simulink model "GuidanceSimV3"  (R2024b)
settings: Solver=VariableStepAuto  StartTime=0.0  StopTime=inf  FixedStep=0.05  RelTol=1e-3
values from neighbouring files (symbols this model uses):
  a_max = 10    [GuidanceSimParams.m]
  a_min = -10    [GuidanceSimParams.m]
  gM = asin(2/3*sin(gT-LOS))+LOS    [GuidanceSimParams.m]
  N = 3.5    [GuidanceSimParams.m]
  Rlethal = 1    [GuidanceSimParams.m]
  RM = [xM;zM]    [GuidanceSimParams.m]
  RT = [xT;zT]    [GuidanceSimParams.m]
  Vcinit = MS*cos(gM-LOS)-TS*cos(gT-LOS)    [GuidanceSimParams.m]
  VM = [600*cos(gM),-600*sin(gM)]    [GuidanceSimParams.m]
  VT = [400*cos(gT),-400*sin(gT)]    [GuidanceSimParams.m]
  Wn_hom = 7    [GuidanceSimParams.m]
undefined symbols (not defined in the file or in its folder): eta, type
libraries: simulink_extras x2, simulink x2, aerolibanim x1
settings Model: Creator=Ameya  LastModifiedBy=Ameya
settings SolverCC: EnableFixedStepZeroCrossing=on

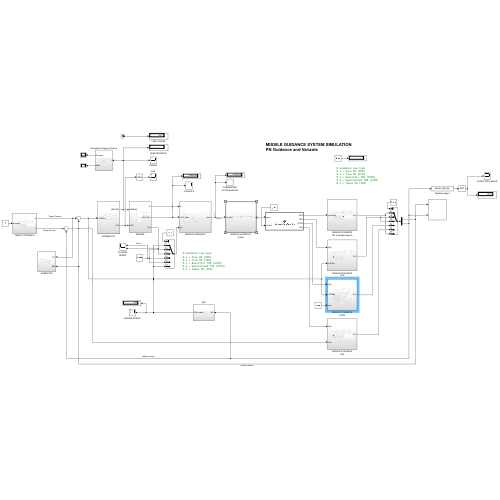
[thumbnail: Simulink's stored preview of the top-level diagram]
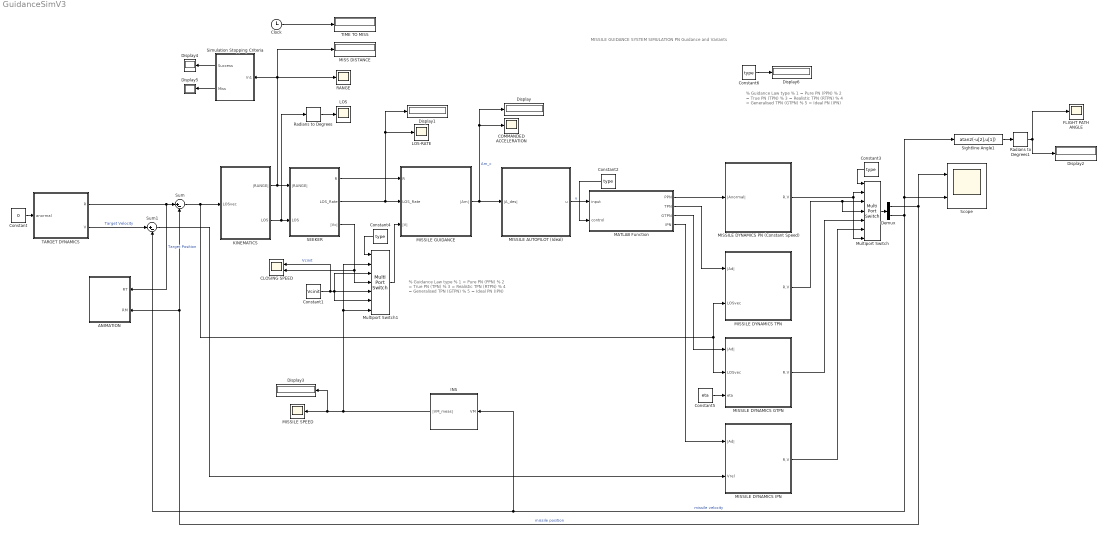
== system GuidanceSimV3 ==
  note: % Guidance Law type
      | % 1 = Pure PN (PPN)
      | % 2 = True PN (TPN)
      | % 3 = Realistic TPN (RTPN)
      | % 4 = Generalised TPN (GTPN)
      | % 5 = Ideal PN (IPN)
  note: MISSILE GUIDANCE SYSTEM SIMULATION
      | PN Guidance and Variants
  note: % Guidance Law type
      | % 1 = Pure PN (PPN)
      | % 2 = True PN (TPN)
      | % 3 = Realistic TPN (RTPN)
      | % 4 = Generalised TPN (GTPN)
      | % 5 = Ideal PN (IPN)
  ANIMATION : Subsystem
  CLOSING SPEED : Scope  NumInputPorts=2
  COMMANDED ACCELERATION : Scope
  Clock : Clock
  Constant : Constant  Value=0
  Constant1 : Constant  Value=Vcinit
  Constant{2..4,6} (4 alike) : Constant  Value=type
  Constant5 : Constant  Value=eta
  Demux : Demux  Outputs=2
  Display{,1..6} (7 alike) : Display
  FLIGHT PATH ANGLE : Scope
  INS : Subsystem
  KINEMATICS : Subsystem
  LOS : Scope
  LOS-RATE : Scope
  MATLAB Function : MATLAB Function  TreatAsAtomicUnit=on
  MISS DISTANCE : Display
  MISSILE AUTOPILOT (Ideal) : Subsystem
  MISSILE DYNAMICS GTPN : Subsystem
  MISSILE DYNAMICS IPN : Subsystem
  MISSILE DYNAMICS PN (Constant Speed) : Subsystem
  MISSILE DYNAMICS TPN : Subsystem
  MISSILE GUIDANCE : Subsystem
  MISSILE SPEED : Scope
  Multiport Switch : MultiPortSwitch  Inputs=5  DataPortForDefault=Additional data port  SaturateOnIntegerOverflow=off  InputSameDT=off
  Multiport Switch1 : MultiPortSwitch  Inputs=5  DataPortForDefault=Additional data port  SaturateOnIntegerOverflow=off  InputSameDT=off
  RANGE : Scope
  Radians to Degrees : simulink_extras/Transformations/Radians to Degrees
  Radians to Degrees1 : simulink_extras/Transformations/Radians to Degrees
  SEEKER : Subsystem
  Scope : Scope  NumInputPorts=2
  Sightline Angle1 : Fcn  Expr=atan2(-u[2],u[1])
  Simulation Stopping Criteria : Subsystem
  Sum : Sum  Inputs=|+-
  Sum1 : Sum  Inputs=|+-
  TARGET DYNAMICS : Subsystem
  TIME TO MISS : Display
  wires:
  MISSILE GUIDANCE/1(|Am|) -> COMMANDED ACCELERATION/1, Display/1, MISSILE AUTOPILOT (Ideal)/1(|A_des|)  "Am_c"
  Constant/1 -> TARGET DYNAMICS/1(anormal)
  Radians to Degrees/1 -> LOS/1
  INS/1(|VM_meas|) -> Display3/1, MISSILE SPEED/1, Multiport Switch1/7, Multiport Switch1/2
  TARGET DYNAMICS/1(R) -> ANIMATION/1(RT), Sum/1  "Target Position"
  Sum/1 -> MISSILE DYNAMICS TPN/2(LOSvec), MISSILE DYNAMICS GTPN/2(LOSvec), KINEMATICS/1(LOSvec)
  KINEMATICS/1(|RANGE|) -> Simulation Stopping Criteria/1(In1), RANGE/1, MISS DISTANCE/1, SEEKER/1(|RANGE|)
  KINEMATICS/2(LOS) -> Radians to Degrees/1, SEEKER/2(LOS)
  SEEKER/2(LOS_Rate) -> Display1/1, LOS-RATE/1, MISSILE GUIDANCE/2(LOS_Rate)
  SEEKER/1(R) -> MISSILE GUIDANCE/1(R)
  Sightline Angle1/1 -> Radians to Degrees1/1
  Radians to Degrees1/1 -> FLIGHT PATH ANGLE/1, Display2/1
  Simulation Stopping Criteria/1(Success) -> Display4/1
  Simulation Stopping Criteria/2(Miss) -> Display5/1
  MISSILE AUTOPILOT (Ideal)/1(u) -> MATLAB Function/1(input)  "u"
  Constant2/1 -> MATLAB Function/2(control)
  MATLAB Function/1(PPN) -> MISSILE DYNAMICS PN (Constant Speed)/1(|Anormal|)
  MATLAB Function/2(TPN) -> MISSILE DYNAMICS TPN/1(|Ad|)
  MATLAB Function/3(GTPN) -> MISSILE DYNAMICS GTPN/1(|Ad|)
  MISSILE DYNAMICS PN (Constant Speed)/1(R,V) -> Multiport Switch/7, Multiport Switch/2
  MISSILE DYNAMICS TPN/1(R,V) -> Multiport Switch/4, Multiport Switch/3
  MISSILE DYNAMICS GTPN/1(R,V) -> Multiport Switch/5
  Constant3/1 -> Multiport Switch/1
  Multiport Switch/1 -> Demux/1
  Demux/1 -> Sum/2, ANIMATION/2(RM), Scope/1  "missile position"
  Demux/2 -> INS/1(VM), Sum1/2, Sightline Angle1/1, Scope/2  "missile velocity"
  MATLAB Function/4(IPN) -> MISSILE DYNAMICS IPN/1(|Ad|)
  TARGET DYNAMICS/2(V) -> Sum1/1  "Target Velocity"
  Sum1/1 -> MISSILE DYNAMICS IPN/2(Vrel)
  MISSILE DYNAMICS IPN/1(R,V) -> Multiport Switch/6
  Multiport Switch1/1 -> MISSILE GUIDANCE/3(|V|)
  Constant1/1 -> CLOSING SPEED/1, Multiport Switch1/3, Multiport Switch1/6, Multiport Switch1/5  "Vcinit"
  SEEKER/3(|Vc|) -> CLOSING SPEED/2, Multiport Switch1/4
  Constant4/1 -> Multiport Switch1/1
  Constant5/1 -> MISSILE DYNAMICS GTPN/3(eta)
  Clock/1 -> TIME TO MISS/1
  Constant6/1 -> Display6/1

== system GuidanceSimV3/ANIMATION ==
  RT : Inport
  RM : Inport  Port=2
  3DoF Animation1 : aerolibanim/3DoF Animation  u1=[0 5000 -2000 2000 -5050 -3]  u2=0.05  u3=1  u5=Fly alongside  u6=[2000 500 -3150]  u7=10  u8=off
  Constant1 : Constant  Value=gM
  wires:
  Constant1/1 -> 3DoF Animation1/3
  RT/1 -> 3DoF Animation1/1
  RM/1 -> 3DoF Animation1/2

== system GuidanceSimV3/INS ==
  VM : Inport
  Dot Product : DotProduct  OutDataTypeStr=Inherit: Inherit via internal rule
  Sqrt : Sqrt
  |VM_meas| : Outport
  wires:
  Dot Product/1 -> Sqrt/1
  Sqrt/1 -> |VM_meas|/1
  VM/1 -> Dot Product/1, Dot Product/2

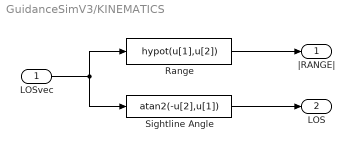
== system GuidanceSimV3/KINEMATICS ==
  LOSvec : Inport
  Range : Fcn  Expr=hypot(u[1],u[2])
  Sightline Angle : Fcn  Expr=atan2(-u[2],u[1])
  |RANGE| : Outport
  LOS : Outport  Port=2
  wires:
  LOSvec/1 -> Range/1, Sightline Angle/1
  Range/1 -> |RANGE|/1
  Sightline Angle/1 -> LOS/1

== system GuidanceSimV3/MISSILE AUTOPILOT (Ideal) ==
  |A_des| : Inport
  Gain : Gain
  u : Outport
  wires:
  |A_des|/1 -> Gain/1
  Gain/1 -> u/1

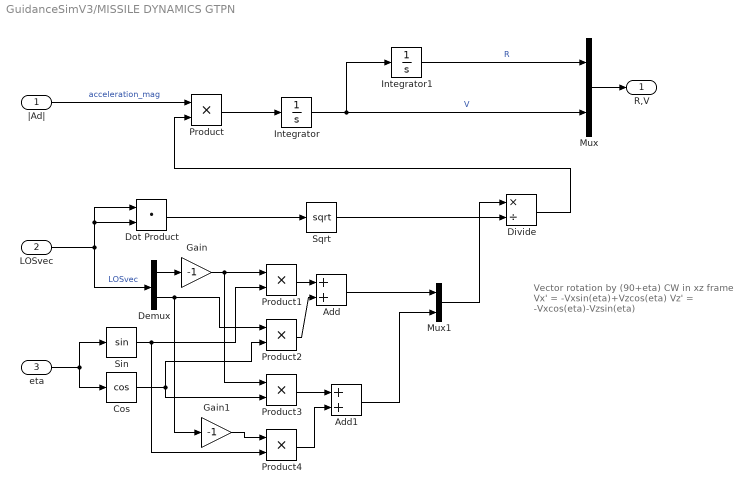
== system GuidanceSimV3/MISSILE DYNAMICS GTPN ==
  note: Vector rotation by (90+eta) CW in xz frame
      | Vx' = -Vxsin(eta)+Vzcos(eta)
      | Vz' = -Vxcos(eta)-Vzsin(eta)
  |Ad| : Inport
  LOSvec : Inport  Port=2
  eta : Inport  Port=3
  Add : Sum
  Add1 : Sum
  Cos : Trigonometry  Operator=cos
  Demux : Demux  Outputs=2
  Divide : Product  Inputs=*/
  Dot Product : DotProduct  OutDataTypeStr=Inherit: Inherit via internal rule
  Gain : Gain  Gain=-1
  Gain1 : Gain  Gain=-1
  Integrator : Integrator  InitialCondition=VM
  Integrator1 : Integrator  InitialCondition=RM
  Mux : Mux  Inputs=2
  Mux1 : Mux  Inputs=2
  Product{,1..4} (5 alike) : Product
  Sin : Trigonometry
  Sqrt : Sqrt
  R,V : Outport
  wires:
  |Ad|/1 -> Product/1  "acceleration_mag"
  Dot Product/1 -> Sqrt/1
  Demux/1 -> Gain/1
  Sqrt/1 -> Divide/2
  Divide/1 -> Product/2
  Mux1/1 -> Divide/1
  Product/1 -> Integrator/1
  Integrator/1 -> Integrator1/1, Mux/2  "V"
  LOSvec/1 -> Demux/1, Dot Product/2, Dot Product/1  "LOSvec"
  Mux/1 -> R,V/1
  Integrator1/1 -> Mux/1  "R"
  eta/1 -> Cos/1, Sin/1
  Gain/1 -> Product3/1, Product1/1
  Sin/1 -> Product4/2, Product1/2
  Product1/1 -> Add/1
  Add/1 -> Mux1/1
  Product2/1 -> Add/2
  Demux/2 -> Gain1/1, Product2/1
  Cos/1 -> Product2/2, Product3/2
  Product3/1 -> Add1/1
  Gain1/1 -> Product4/1
  Product4/1 -> Add1/2
  Add1/1 -> Mux1/2

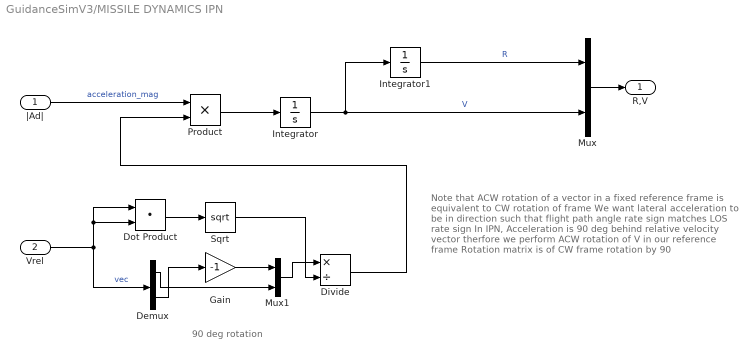
== system GuidanceSimV3/MISSILE DYNAMICS IPN ==
  note: Note that ACW rotation of a vector in
      | a fixed reference frame is equivalent to
      | CW rotation of frame
      |
      | We want lateral acceleration to be in direction
      | such that flight path angle rate sign matches LOS rate sign
      | In IPN, Acceleration is 90 deg behind relative velocity vector
      | therfore we perform ACW rotation of V in our reference frame
      | Rotation matrix is of CW frame rotation by 90
  note: 90 deg rotation
  |Ad| : Inport
  Vrel : Inport  Port=2
  Demux : Demux  Outputs=2
  Divide : Product  Inputs=*/
  Dot Product : DotProduct  OutDataTypeStr=Inherit: Inherit via internal rule
  Gain : Gain  Gain=-1
  Integrator : Integrator  InitialCondition=VM
  Integrator1 : Integrator  InitialCondition=RM
  Mux : Mux  Inputs=2
  Mux1 : Mux  Inputs=2
  Product : Product
  Sqrt : Sqrt
  R,V : Outport
  wires:
  |Ad|/1 -> Product/1  "acceleration_mag"
  Demux/2 -> Gain/1
  Dot Product/1 -> Sqrt/1
  Sqrt/1 -> Divide/2
  Divide/1 -> Product/2
  Mux1/1 -> Divide/1
  Demux/1 -> Mux1/2
  Product/1 -> Integrator/1
  Integrator/1 -> Integrator1/1, Mux/2  "V"
  Vrel/1 -> Demux/1, Dot Product/2, Dot Product/1  "vec"
  Mux/1 -> R,V/1
  Integrator1/1 -> Mux/1  "R"
  Gain/1 -> Mux1/1

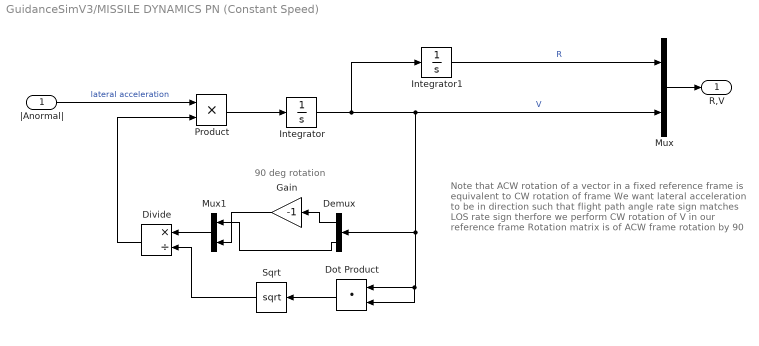
== system GuidanceSimV3/MISSILE DYNAMICS PN (Constant Speed) ==
  note: 90 deg rotation
  note: Note that ACW rotation of a vector in
      | a fixed reference frame is equivalent to
      | CW rotation of frame
      |
      | We want lateral acceleration to be in direction
      | such that flight path angle rate sign matches LOS rate sign
      | therfore we perform CW rotation of V in our reference frame
      | Rotation matrix is of ACW frame rotation by 90
  |Anormal| : Inport
  Demux : Demux  Outputs=2
  Divide : Product  Inputs=*/
  Dot Product : DotProduct  OutDataTypeStr=Inherit: Inherit via internal rule
  Gain : Gain  Gain=-1
  Integrator : Integrator  InitialCondition=VM
  Integrator1 : Integrator  InitialCondition=RM
  Mux : Mux  Inputs=2
  Mux1 : Mux  Inputs=2
  Product : Product
  Sqrt : Sqrt
  R,V : Outport
  wires:
  |Anormal|/1 -> Product/1  "lateral acceleration"
  Integrator1/1 -> Mux/1  "R"
  Demux/2 -> Mux1/1
  Dot Product/1 -> Sqrt/1
  Demux/1 -> Gain/1
  Sqrt/1 -> Divide/2
  Divide/1 -> Product/2
  Mux1/1 -> Divide/1
  Gain/1 -> Mux1/2
  Product/1 -> Integrator/1
  Integrator/1 -> Integrator1/1, Mux/2, Dot Product/2, Dot Product/1, Demux/1  "V"
  Mux/1 -> R,V/1

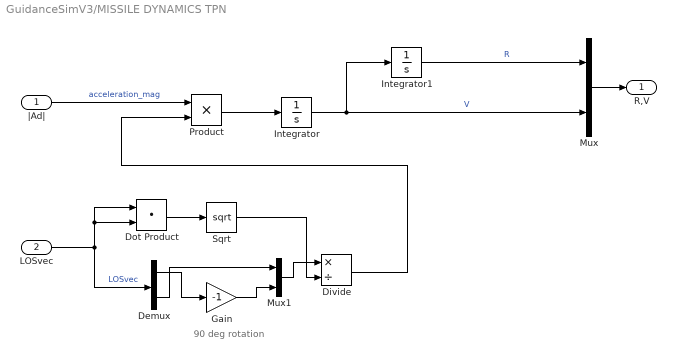
== system GuidanceSimV3/MISSILE DYNAMICS TPN ==
  note: 90 deg rotation
  |Ad| : Inport
  LOSvec : Inport  Port=2
  Demux : Demux  Outputs=2
  Divide : Product  Inputs=*/
  Dot Product : DotProduct  OutDataTypeStr=Inherit: Inherit via internal rule
  Gain : Gain  Gain=-1
  Integrator : Integrator  InitialCondition=VM
  Integrator1 : Integrator  InitialCondition=RM
  Mux : Mux  Inputs=2
  Mux1 : Mux  Inputs=2
  Product : Product
  Sqrt : Sqrt
  R,V : Outport
  wires:
  |Ad|/1 -> Product/1  "acceleration_mag"
  Demux/2 -> Mux1/1
  Dot Product/1 -> Sqrt/1
  Demux/1 -> Gain/1
  Sqrt/1 -> Divide/2
  Divide/1 -> Product/2
  Mux1/1 -> Divide/1
  Gain/1 -> Mux1/2
  Product/1 -> Integrator/1
  Integrator/1 -> Integrator1/1, Mux/2  "V"
  LOSvec/1 -> Demux/1, Dot Product/2, Dot Product/1  "LOSvec"
  Mux/1 -> R,V/1
  Integrator1/1 -> Mux/1  "R"

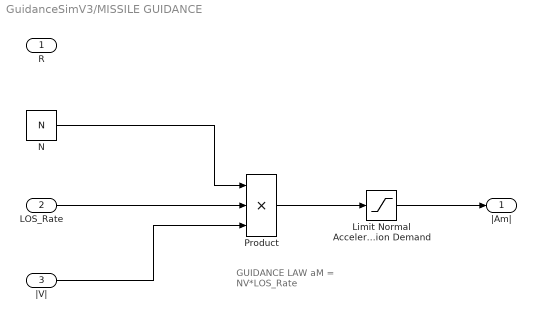
== system GuidanceSimV3/MISSILE GUIDANCE ==
  note: GUIDANCE LAW
      | aM = NV*LOS_Rate
  R : Inport
  LOS_Rate : Inport  Port=2
  |V| : Inport  Port=3
  Limit Normal Acceleration Demand : Saturate  UpperLimit=a_max+100  LowerLimit=a_min
  N : Constant  Value=N
  Product : Product  Inputs=3
  |Am| : Outport
  wires:
  N/1 -> Product/1
  Product/1 -> Limit Normal Acceleration Demand/1
  LOS_Rate/1 -> Product/2
  |V|/1 -> Product/3
  Limit Normal Acceleration Demand/1 -> |Am|/1

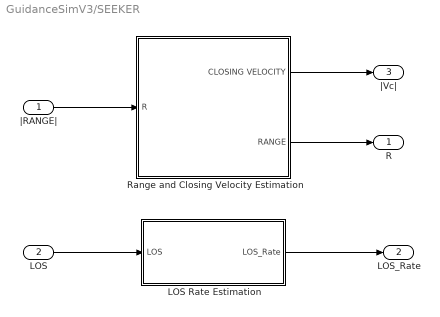
== system GuidanceSimV3/SEEKER ==
  |RANGE| : Inport
  LOS : Inport  Port=2
  LOS Rate Estimation : Subsystem
  Range and Closing Velocity Estimation : Subsystem
  R : Outport  InitialOutput=0  VectorParamsAs1DForOutWhenUnconnected=off
  LOS_Rate : Outport  Port=2
  |Vc| : Outport  Port=3  InitialOutput=0  VectorParamsAs1DForOutWhenUnconnected=off
  wires:
  |RANGE|/1 -> Range and Closing Velocity Estimation/1(R)
  Range and Closing Velocity Estimation/1(CLOSING VELOCITY) -> |Vc|/1
  Range and Closing Velocity Estimation/2(RANGE) -> R/1
  LOS/1 -> LOS Rate Estimation/1(LOS)
  LOS Rate Estimation/1(LOS_Rate) -> LOS_Rate/1

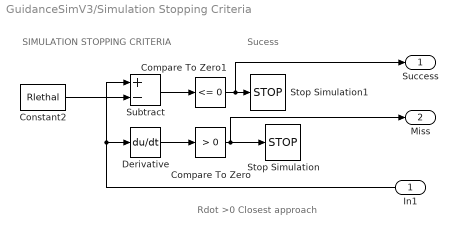
== system GuidanceSimV3/Simulation Stopping Criteria ==
  note: Rdot >0
      | Closest approach
  note: SIMULATION STOPPING CRITERIA
  note: Sucess
  In1 : Inport
  Compare To Zero : simulink/Logic and Bit Operations/Compare To Zero  relop=>  OutDataTypeStr=boolean
  Compare To Zero1 : simulink/Logic and Bit Operations/Compare To Zero  relop=<=  OutDataTypeStr=boolean
  Constant2 : Constant  Value=Rlethal
  Derivative : Derivative
  Stop Simulation : Stop
  Stop Simulation1 : Stop
  Subtract : Sum  Inputs=+-
  Success : Outport
  Miss : Outport  Port=2
  wires:
  Derivative/1 -> Compare To Zero/1
  Compare To Zero1/1 -> Success/1, Stop Simulation1/1
  In1/1 -> Derivative/1, Subtract/1
  Compare To Zero/1 -> Miss/1, Stop Simulation/1
  Subtract/1 -> Compare To Zero1/1
  Constant2/1 -> Subtract/2

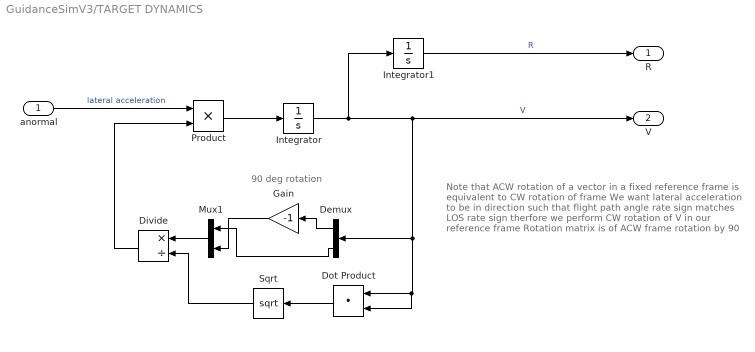
== system GuidanceSimV3/TARGET DYNAMICS ==
  note: 90 deg rotation
  note: Note that ACW rotation of a vector in
      | a fixed reference frame is equivalent to
      | CW rotation of frame
      |
      | We want lateral acceleration to be in direction
      | such that flight path angle rate sign matches LOS rate sign
      | therfore we perform CW rotation of V in our reference frame
      | Rotation matrix is of ACW frame rotation by 90
  anormal : Inport
  Demux : Demux  Outputs=2
  Divide : Product  Inputs=*/
  Dot Product : DotProduct  OutDataTypeStr=Inherit: Inherit via internal rule
  Gain : Gain  Gain=-1
  Integrator : Integrator  InitialCondition=VT
  Integrator1 : Integrator  InitialCondition=RT
  Mux1 : Mux  Inputs=2
  Product : Product
  Sqrt : Sqrt
  R : Outport
  V : Outport  Port=2
  wires:
  anormal/1 -> Product/1  "lateral acceleration"
  Integrator1/1 -> R/1  "R"
  Demux/2 -> Mux1/1
  Dot Product/1 -> Sqrt/1
  Demux/1 -> Gain/1
  Sqrt/1 -> Divide/2
  Divide/1 -> Product/2
  Mux1/1 -> Divide/1
  Gain/1 -> Mux1/2
  Product/1 -> Integrator/1
  Integrator/1 -> Integrator1/1, V/1, Dot Product/2, Dot Product/1, Demux/1  "V"

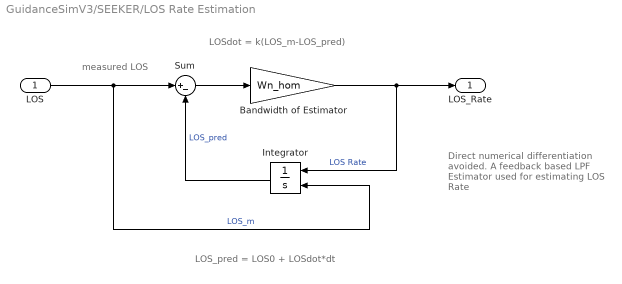
== system GuidanceSimV3/SEEKER/LOS Rate Estimation ==
  note: LOS_pred = LOS0 + LOSdot*dt
  note: LOSdot = k(LOS_m-LOS_pred)
  note: measured LOS
  note: Direct numerical differentiation avoided.
      | A feedback based LPF Estimator used for estimating LOS Rate
  LOS : Inport
  Bandwidth of Estimator : Gain  Gain=Wn_hom  SaturateOnIntegerOverflow=on  OutDataTypeStr=Inherit: Same as input  ParamDataTypeStr=Inherit: Same as input
  Integrator : Integrator  InitialConditionSource=external
  Sum : Sum  Inputs=|+-
  LOS_Rate : Outport
  wires:
  LOS/1 -> Sum/1, Integrator/2  "LOS_m"
  Sum/1 -> Bandwidth of Estimator/1
  Bandwidth of Estimator/1 -> Integrator/1, LOS_Rate/1  "LOS Rate"
  Integrator/1 -> Sum/2  "LOS_pred"

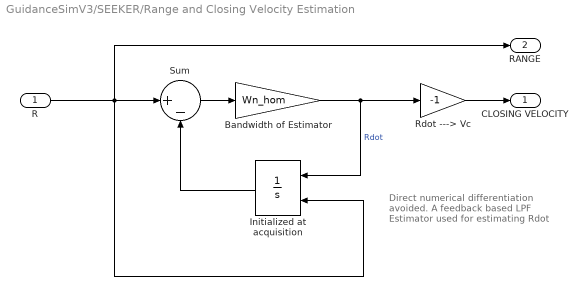
== system GuidanceSimV3/SEEKER/Range and Closing Velocity Estimation ==
  note: Direct numerical differentiation avoided.
      | A feedback based LPF Estimator used for estimating Rdot
  R : Inport
  Bandwidth of Estimator : Gain  Gain=Wn_hom  SaturateOnIntegerOverflow=on  OutDataTypeStr=Inherit: Same as input  ParamDataTypeStr=Inherit: Same as input
  Initialized at acquisition : Integrator  InitialConditionSource=external
  Rdot ---> Vc : Gain  Gain=-1  SaturateOnIntegerOverflow=on  OutDataTypeStr=Inherit: Same as input  ParamDataTypeStr=Inherit: Same as input
  Sum : Sum  Inputs=|+-  InputSameDT=on  SaturateOnIntegerOverflow=on  OutDataTypeStr=Inherit: Same as first input
  CLOSING VELOCITY : Outport  InitialOutput=0  VectorParamsAs1DForOutWhenUnconnected=off
  RANGE : Outport  Port=2  InitialOutput=0  VectorParamsAs1DForOutWhenUnconnected=off
  wires:
  R/1 -> Sum/1, Initialized at acquisition/2, RANGE/1
  Initialized at acquisition/1 -> Sum/2
  Bandwidth of Estimator/1 -> Rdot ---> Vc/1, Initialized at acquisition/1  "Rdot"
  Rdot ---> Vc/1 -> CLOSING VELOCITY/1
  Sum/1 -> Bandwidth of Estimator/1

== matlab function GuidanceSimV3/MATLAB Function ==
  data: input input; PPN output; control input; TPN output; GTPN output; IPN output
function [PPN, TPN, GTPN, IPN] = guidanceLawSelector(input, control)
    PPN = 0; TPN = 0; GTPN = 0; IPN = 0;
    if control == 1
        PPN = input;
    elseif control == 2||control == 3
        TPN = input;
    elseif control == 4
        GTPN = input;
    elseif control == 5
        IPN = input;
    end
end
